simulink model "simModel2020"  (R2023b)
settings: Solver=ode4  StartTime=0  StopTime=360  FixedStep=0.01  RelTol=1e-3
values from neighbouring files (symbols this model uses):
  B747 =     [B747.mat]
undefined symbols (not defined in the file or in its folder): airport, APP, control, Curise, Earth, env, ft, m, navData, navParam, Newton, plotTrack, Raphson, s, TakeOff, WGS84
libraries: aerolibconvert2 x18, simulink x15, sharedtransform x4, aerolibfltsims x3, aerolibatmos2 x2, shared6dof x2, aerolibasang x2, dspsrcs4 x2, aerolibwind2 x2, aerolibanimutils x1, aerolibpropulsion2 x1, aerolibtransform2 x1
(part 4 of 6)

== system simModel2020/AutoPilot/InnerLoopAutopilot/Longitudinal Channel经度通道/AutoThrottle/AT Mode = 3,Throttle Control/Filter1 ==
  x : Inport
  SW_x(k-1) : Inport  Port=2
  time : Inport  Port=3
  Constant : Constant  SampleTime=-1
  Data Type Conversion3 : DataTypeConversion  SaturateOnIntegerOverflow=off  RndMeth=Floor
  Detect Change : simulink/Logic and Bit Operations/Detect Change  vinit=0  OutDataTypeStr=boolean
  Gain : Gain  Gain=0.5
  Math Function : Math  SignedPower=on
  Product : Product
  Product1 : Product
  Subsystem : Subsystem
      mask Display: disp('S/H')
  Sum : Sum  Inputs=|+-
  Sum1 : Sum  Inputs=|++
  Sum2 : Sum  Inputs=+-|
  y : Outport
  wires:
  Product/1 -> Sum1/2
  SW_x(k-1)/1 -> Product/2
  Product1/1 -> Sum1/1
  x/1 -> Product1/1
  Sum1/1 -> Data Type Conversion3/1
  time/1 -> Subsystem/1(In), Sum2/2
  Subsystem/1(" ") -> Sum2/1
  Sum2/1 -> Gain/1
  Gain/1 -> Math Function/1
  Math Function/1 -> Sum/2, Product/1
  Sum/1 -> Product1/2
  Data Type Conversion3/1 -> y/1
  Constant/1 -> Detect Change/1, Sum/1
  Detect Change/1 -> Subsystem/Enable

== system simModel2020/AutoPilot/InnerLoopAutopilot/Longitudinal Channel经度通道/AutoThrottle/AT Mode = 5,Idle/Filter1 ==
  x : Inport
  SW_x(k-1) : Inport  Port=2
  time : Inport  Port=3
  Constant : Constant  SampleTime=-1
  Data Type Conversion3 : DataTypeConversion  SaturateOnIntegerOverflow=off  RndMeth=Floor
  Detect Change : simulink/Logic and Bit Operations/Detect Change  vinit=0  OutDataTypeStr=boolean
  Gain : Gain  Gain=0.5
  Math Function : Math  SignedPower=on
  Product : Product
  Product1 : Product
  Subsystem : Subsystem
      mask Display: disp('S/H')
  Sum : Sum  Inputs=|+-
  Sum1 : Sum  Inputs=|++
  Sum2 : Sum  Inputs=+-|
  y : Outport
  wires:
  Product/1 -> Sum1/2
  SW_x(k-1)/1 -> Product/2
  Product1/1 -> Sum1/1
  x/1 -> Product1/1
  Sum1/1 -> Data Type Conversion3/1
  time/1 -> Subsystem/1(In), Sum2/2
  Subsystem/1(" ") -> Sum2/1
  Sum2/1 -> Gain/1
  Gain/1 -> Math Function/1
  Math Function/1 -> Sum/2, Product/1
  Sum/1 -> Product1/2
  Data Type Conversion3/1 -> y/1
  Constant/1 -> Detect Change/1, Sum/1
  Detect Change/1 -> Subsystem/Enable

== system simModel2020/AutoPilot/InnerLoopAutopilot/Longitudinal Channel经度通道/AutoThrottle/AT Mode = 5,Idle/Rate Limiter Dynamic with External IC and Autoreset for Change in IC ==
  note: Y(k)
  note: U(k)
  up : Inport
  u : Inport  Port=2
  lo : Inport  Port=3
  IC : Inport  Port=4
  Abs : Abs  SaturateOnIntegerOverflow=off
  Delay : Delay  DelayLength=1
  Difference Inputs1 : Sum  Description=Add in CPU  DisableCoverage=on  Inputs=+-  OutDataTypeStr=Inherit: Inherit via back propagation
  Difference Inputs2 : Sum  Description=Add in CPU  OutDataTypeStr=Inherit: Inherit via back propagation
  Saturation Dynamic : Subsystem  mask(Saturation Dynamic){OutMin=[], OutMax=[], OutDataTypeStr=Inherit: Same as second input, OutputDataTypeScalingMode=Same as second input, OutDataType=fixdt(1, 16), OutScaling=2^-10, LockScale=off, RndMeth=Floor, DoSatur=off}
      mask prompts: OutMin "Simulink:masks:OutputMinimum_MP"; OutMax "Simulink:masks:OutputMaximum_MP"; OutDataTypeStr "Simulink:masks:OutputDataType_MP"; OutputDataTypeScalingMode "Simulink:masks:OutputDataTypeMode_MP"; OutDataType "Simulink:masks:OutputDataTypeegFixdt116Fixdtsingle_MP"; OutScaling "Simulink:masks:OutputScalingSlopeEg29OrSlopeBias_MP"; LockScale "Simulink:masks:LockOutputDataTypeAgainstFxpTools_MP"; RndMeth "Simulink:masks:IntegerRoundingMode_MP"; DoSatur "Simulink:masks:SaturateOnIntegerOverflow_MP"
      mask help: Simulink:masks:SaturationDynamic_MD
      mask init: same as simModel2020/AutoPilot/InnerLoopAutopilot/Longitudinal Channel经度通道/AutoThrottle/AT Mode = 0,Recycle/Rate Limiter Dynamic with External IC and Autoreset for Change in IC/Saturation Dynamic
      mask Callback OutDataTypeStr: fixptdialog(gcbh)
      mask TypeOptions OutputDataTypeScalingMode: double | single | int8 | uint8 | int16 | uint16 | int32 | uint32 | Specify via dialog | Same as second input
      mask Callback OutputDataTypeScalingMode: fixptdialog(gcbh)
      mask Callback OutDataType: fixptdialog(gcbh)
      mask TypeOptions RndMeth: Simulink:masks:Ceiling | Simulink:masks:Convergent | Simulink:masks:Floor | Simulink:masks:Nearest | Simulink:masks:Round | Simulink:masks:Simplest | Simulink:masks:Zero
  Subsystem : Subsystem
  Subtract : Sum  Inputs=+-
  Unit Delay Resettable External IC : Subsystem  mask(Unit Delay Resettable External Initial Condition){tsamp=-1}
      mask prompts: tsamp "Simulink:masks:SampleTime_MP"
      mask help: Simulink:masks:UnitDelayResettableExternalInitialCondition_MD
      mask Display: dpoly(1,[1 0],'z')
  delta fall limit : Product  DisableCoverage=on  Inputs=**  OutDataTypeStr=Inherit: Inherit via back propagation  SaturateOnIntegerOverflow=on
  delta rise limit : Product  DisableCoverage=on  Inputs=**  OutDataTypeStr=Inherit: Inherit via back propagation  SaturateOnIntegerOverflow=on
  sample time : SampleTimeMath  DisableCoverage=on  TsampMathOp=Ts Only  weightValue=1
  Y : Outport
  wires:
  Abs/1 -> Subsystem/1(WP Fly)
  Subsystem/1(Just Enab) -> Unit Delay Resettable External IC/2(R)
  Subtract/1 -> Abs/1
  Delay/1 -> Subtract/1
  sample time/1 -> delta fall limit/2, delta rise limit/2
  lo/1 -> delta fall limit/1
  delta rise limit/1 -> Saturation Dynamic/1(up)
  up/1 -> delta rise limit/1
  Difference Inputs2/1 -> Unit Delay Resettable External IC/1(u), Y/1
  Unit Delay Resettable External IC/1(y) -> Difference Inputs1/2, Difference Inputs2/2  "Y(k-1)"
  Saturation Dynamic/1(y) -> Difference Inputs2/1
  delta fall limit/1 -> Saturation Dynamic/3(lo)
  u/1 -> Difference Inputs1/1, sample time/1
  Difference Inputs1/1 -> Saturation Dynamic/2(u)  "( U(k) - Y(k-1) )"
  IC/1 -> Delay/1, Unit Delay Resettable External IC/3(IC), Subtract/2

== system simModel2020/AutoPilot/InnerLoopAutopilot/Longitudinal Channel经度通道/AutoThrottle/Sample(1//z)/Detect Change ==
  note: Edge
  note: U(k)
  U : Inport
  Delay Input1 : UnitDelay  Description=Store in Global RAM  DisableCoverage=on  InitialCondition=vinit  SampleTime=-1  HasFrameUpgradeWarning=on
  FixPt Relational Operator : RelationalOperator  Operator=~=  OutDataTypeStr=boolean  ZeroCross=off  InputSameDT=off
  Y : Outport  InitialOutput=0
  wires:
  FixPt Relational Operator/1 -> Y/1
  Delay Input1/1 -> FixPt Relational Operator/2  "U(k-1)"
  U/1 -> FixPt Relational Operator/1, Delay Input1/1

== system simModel2020/AutoPilot/InnerLoopAutopilot/Longitudinal Channel经度通道/AutoThrottle/Sample(1//z)/Sample and Hold ==
  In : Inport
  Trigger : TriggerPort  TriggerType=either  VariantControl=Variant  ZeroCross=off
  " " : Outport  InitialOutput=initCond
  wires:
  In/1 -> " "/1

== system simModel2020/AutoPilot/InnerLoopAutopilot/Longitudinal Channel经度通道/PitchStyle/Altitude Hold/Filter1 ==
  x : Inport
  SW_x(k-1) : Inport  Port=2
  time : Inport  Port=3
  Constant : Constant  SampleTime=-1
  Data Type Conversion : DataTypeConversion  SaturateOnIntegerOverflow=off  RndMeth=Floor
  Detect Change : simulink/Logic and Bit Operations/Detect Change  vinit=0  OutDataTypeStr=boolean
  Gain : Gain  Gain=0.5
  Math Function : Math  SignedPower=on
  Product : Product
  Product1 : Product
  Subsystem : Subsystem
      mask Display: disp('S/H')
  Sum : Sum  Inputs=|+-
  Sum1 : Sum  Inputs=|++
  Sum2 : Sum  Inputs=+-|
  y : Outport
  wires:
  Product/1 -> Sum1/2
  SW_x(k-1)/1 -> Product/2
  Product1/1 -> Sum1/1
  x/1 -> Product1/1
  Sum1/1 -> Data Type Conversion/1
  time/1 -> Subsystem/1(In), Sum2/2
  Subsystem/1(" ") -> Sum2/1
  Sum2/1 -> Gain/1
  Gain/1 -> Math Function/1
  Math Function/1 -> Product/1, Sum/2
  Sum/1 -> Product1/2
  Data Type Conversion/1 -> y/1
  Constant/1 -> Sum/1, Detect Change/1
  Detect Change/1 -> Subsystem/Enable

== system simModel2020/AutoPilot/InnerLoopAutopilot/Longitudinal Channel经度通道/PitchStyle/IAS_Control_dE/Filter2 ==
  x : Inport
  SW_x(k-1) : Inport  Port=2
  time : Inport  Port=3
  Constant : Constant  SampleTime=-1
  Data Type Conversion3 : DataTypeConversion  SaturateOnIntegerOverflow=off  RndMeth=Floor
  Detect Change : simulink/Logic and Bit Operations/Detect Change  vinit=0  OutDataTypeStr=boolean
  Gain : Gain  Gain=0.5
  Math Function : Math  SignedPower=on
  Product : Product
  Product1 : Product
  Subsystem : Subsystem
      mask Display: disp('S/H')
  Sum : Sum  Inputs=|+-
  Sum1 : Sum  Inputs=|++
  Sum2 : Sum  Inputs=+-|
  y : Outport
  wires:
  Product/1 -> Sum1/2
  SW_x(k-1)/1 -> Product/2
  Product1/1 -> Sum1/1
  x/1 -> Product1/1
  Sum1/1 -> Data Type Conversion3/1
  time/1 -> Subsystem/1(In), Sum2/2
  Subsystem/1(" ") -> Sum2/1
  Sum2/1 -> Gain/1
  Gain/1 -> Math Function/1
  Math Function/1 -> Sum/2, Product/1
  Sum/1 -> Product1/2
  Data Type Conversion3/1 -> y/1
  Constant/1 -> Detect Change/1, Sum/1
  Detect Change/1 -> Subsystem/Enable

== system simModel2020/AutoPilot/InnerLoopAutopilot/Longitudinal Channel经度通道/PitchStyle/Pitch Control/Compute Feed Forward ==
  dEFFGain : Inport
  Roll : Inport  Port=2
  Add5 : Sum  Inputs=+-  OutDataTypeStr=single
  Constant2 : Constant  OutDataTypeStr=single
      settings: AttributesFormatString=%<Value>
  Constant4 : Constant  OutDataTypeStr=single
      settings: AttributesFormatString=%<Value>
  Product : Product  Inputs=*/  RndMeth=Zero
  Product1 : Product  RndMeth=Zero
  Saturation : Saturate  UpperLimit=pi/3  LowerLimit=-pi/3  OutDataTypeStr=double
  Trigonometric Function : Trigonometry  Operator=cos
  FF : Outport
  wires:
  Product/1 -> Add5/1
  Constant4/1 -> Product/1
  Roll/1 -> Saturation/1
  Trigonometric Function/1 -> Product/2
  Constant2/1 -> Add5/2
  Product1/1 -> FF/1
  Add5/1 -> Product1/2
  Saturation/1 -> Trigonometric Function/1
  dEFFGain/1 -> Product1/1

== system simModel2020/AutoPilot/InnerLoopAutopilot/Longitudinal Channel经度通道/PitchStyle/Pitch Control/Filter2 ==
  x : Inport
  SW_x(k-1) : Inport  Port=2
  time : Inport  Port=3
  Constant : Constant  SampleTime=-1
  Data Type Conversion3 : DataTypeConversion  SaturateOnIntegerOverflow=off  RndMeth=Floor
  Detect Change : simulink/Logic and Bit Operations/Detect Change  vinit=0  OutDataTypeStr=boolean
  Gain : Gain  Gain=0.5
  Math Function : Math  SignedPower=on
  Product : Product
  Product1 : Product
  Subsystem : Subsystem
      mask Display: disp('S/H')
  Sum : Sum  Inputs=|+-
  Sum1 : Sum  Inputs=|++
  Sum2 : Sum  Inputs=+-|
  y : Outport
  wires:
  Product/1 -> Sum1/2
  SW_x(k-1)/1 -> Product/2
  Product1/1 -> Sum1/1
  x/1 -> Product1/1
  Sum1/1 -> Data Type Conversion3/1
  time/1 -> Subsystem/1(In), Sum2/2
  Subsystem/1(" ") -> Sum2/1
  Sum2/1 -> Gain/1
  Gain/1 -> Math Function/1
  Math Function/1 -> Sum/2, Product/1
  Sum/1 -> Product1/2
  Data Type Conversion3/1 -> y/1
  Constant/1 -> Detect Change/1, Sum/1
  Detect Change/1 -> Subsystem/Enable

== system simModel2020/AutoPilot/InnerLoopAutopilot/Longitudinal Channel经度通道/PitchStyle/Rate Limiter Dynamic/Rate Limiter Dynamic with External IC and Autoreset for Change in IC1 ==
  note: U(k)
  note: Y(k)
  up : Inport
  u : Inport  Port=2
  lo : Inport  Port=3
  IC : Inport  Port=4
  Abs : Abs  SaturateOnIntegerOverflow=off
  Delay : Delay  DelayLength=1
  Difference Inputs1 : Sum  Description=Add in CPU  DisableCoverage=on  Inputs=+-  OutDataTypeStr=Inherit: Inherit via back propagation
  Difference Inputs2 : Sum  Description=Add in CPU  OutDataTypeStr=Inherit: Inherit via back propagation
  Saturation Dynamic : Subsystem  mask(Saturation Dynamic){OutMin=[], OutMax=[], OutDataTypeStr=Inherit: Same as second input, OutputDataTypeScalingMode=Same as second input, OutDataType=fixdt(1, 16), OutScaling=2^-10, LockScale=off, RndMeth=Floor, DoSatur=off}
      mask prompts: OutMin "Simulink:masks:OutputMinimum_MP"; OutMax "Simulink:masks:OutputMaximum_MP"; OutDataTypeStr "Simulink:masks:OutputDataType_MP"; OutputDataTypeScalingMode "Simulink:masks:OutputDataTypeMode_MP"; OutDataType "Simulink:masks:OutputDataTypeegFixdt116Fixdtsingle_MP"; OutScaling "Simulink:masks:OutputScalingSlopeEg29OrSlopeBias_MP"; LockScale "Simulink:masks:LockOutputDataTypeAgainstFxpTools_MP"; RndMeth "Simulink:masks:IntegerRoundingMode_MP"; DoSatur "Simulink:masks:SaturateOnIntegerOverflow_MP"
      mask help: Simulink:masks:SaturationDynamic_MD
      mask init: same as simModel2020/AutoPilot/InnerLoopAutopilot/Longitudinal Channel经度通道/AutoThrottle/AT Mode = 0,Recycle/Rate Limiter Dynamic with External IC and Autoreset for Change in IC/Saturation Dynamic
      mask Callback OutDataTypeStr: fixptdialog(gcbh)
      mask TypeOptions OutputDataTypeScalingMode: double | single | int8 | uint8 | int16 | uint16 | int32 | uint32 | Specify via dialog | Same as second input
      mask Callback OutputDataTypeScalingMode: fixptdialog(gcbh)
      mask Callback OutDataType: fixptdialog(gcbh)
      mask TypeOptions RndMeth: Simulink:masks:Ceiling | Simulink:masks:Convergent | Simulink:masks:Floor | Simulink:masks:Nearest | Simulink:masks:Round | Simulink:masks:Simplest | Simulink:masks:Zero
  Subsystem : Subsystem
  Subtract : Sum  Inputs=+-
  Unit Delay Resettable External IC : Subsystem  mask(Unit Delay Resettable External Initial Condition){tsamp=-1}
      mask prompts: tsamp "Simulink:masks:SampleTime_MP"
      mask help: Simulink:masks:UnitDelayResettableExternalInitialCondition_MD
      mask Display: dpoly(1,[1 0],'z')
  Weighted Sample Time : SampleTimeMath  TsampMathOp=Ts Only
  delta fall limit : Product  DisableCoverage=on  Inputs=**  OutDataTypeStr=Inherit: Inherit via back propagation  SaturateOnIntegerOverflow=on
  delta rise limit : Product  DisableCoverage=on  Inputs=**  OutDataTypeStr=Inherit: Inherit via back propagation  SaturateOnIntegerOverflow=on
  Y : Outport
  wires:
  IC/1 -> Subtract/2, Unit Delay Resettable External IC/3(IC), Delay/1
  Difference Inputs1/1 -> Saturation Dynamic/2(u)  "( U(k) - Y(k-1) )"
  u/1 -> Difference Inputs1/1, Weighted Sample Time/1
  delta fall limit/1 -> Saturation Dynamic/3(lo)
  Saturation Dynamic/1(y) -> Difference Inputs2/1
  Unit Delay Resettable External IC/1(y) -> Difference Inputs2/2, Difference Inputs1/2  "Y(k-1)"
  Difference Inputs2/1 -> Y/1, Unit Delay Resettable External IC/1(u)
  up/1 -> delta rise limit/1
  delta rise limit/1 -> Saturation Dynamic/1(up)
  lo/1 -> delta fall limit/1
  Weighted Sample Time/1 -> delta rise limit/2, delta fall limit/2
  Delay/1 -> Subtract/1
  Subtract/1 -> Abs/1
  Subsystem/1(Just Enab) -> Unit Delay Resettable External IC/2(R)
  Abs/1 -> Subsystem/1(WP Fly)

== system simModel2020/AutoPilot/InnerLoopAutopilot/Longitudinal Channel经度通道/PitchStyle/Rate Limiter Dynamic/Sample(1//z) ==
  <Test> : Inport
  x : Inport  Port=2
  Detect Change : Subsystem  mask(Detect Change){vinit=0, InputProcessing=Elements as channels (sample based), OutDataTypeStr=boolean}
      mask prompts: vinit "Simulink:masks:InitialCondition_MP"; InputProcessing "Simulink:masks:InputProcessing_MP"; OutDataTypeStr "Simulink:masks:OutputDataType_MP"
      mask help: Simulink:masks:DetectChange_MD
      mask init:
      | initDetectBlocks();
      mask TypeOptions InputProcessing: Simulink:masks:ColumnsAsChannelsFrameBased | Simulink:masks:ElementsAsChannelsSampleBased
      mask TypeOptions OutDataTypeStr: Simulink:masks:uint8 | Simulink:masks:boolean
      mask Display: fprintf('U ~= U/z')
  Sample and Hold : Subsystem  TreatAsAtomicUnit=on  mask(Sample and Hold){trig=Either edge, initCond=0, latchinput=off}
      mask prompts: trig "Trigger type:"; initCond "Initial condition:"; latchinput "Latch (buffer) input"
      mask help: Sample and hold the input signal. If Latch (buffer) input is selected, then this block produces the value of the input from the previous time step.
      mask init: same as simModel2020/AutoPilot/InnerLoopAutopilot/Latitudinal Channel维度通道/Sample(1//z)/Sample and Hold
      mask Help: eval('blocksethelp');
      mask TypeOptions trig: Rising edge | Falling edge | Either edge
      mask Display: disp('S/H')
  y : Outport
  wires:
  <Test>/1 -> Detect Change/1(U)
  Detect Change/1(Y) -> Sample and Hold/Trigger
  x/1 -> Sample and Hold/1(In)
  Sample and Hold/1(" ") -> y/1

== system simModel2020/AutoPilot/InnerLoopAutopilot/Longitudinal Channel经度通道/PitchStyle/Rate Limiter Dynamic1/Rate Limiter Dynamic with External IC and Autoreset for Change in IC ==
  note: Y(k)
  note: U(k)
  up : Inport
  u : Inport  Port=2
  lo : Inport  Port=3
  IC : Inport  Port=4
  Abs : Abs  SaturateOnIntegerOverflow=off
  Delay : Delay  DelayLength=1
  Difference Inputs1 : Sum  Description=Add in CPU  DisableCoverage=on  Inputs=+-  OutDataTypeStr=Inherit: Inherit via back propagation
  Difference Inputs2 : Sum  Description=Add in CPU  OutDataTypeStr=Inherit: Inherit via back propagation
  Saturation Dynamic : Subsystem  mask(Saturation Dynamic){OutMin=[], OutMax=[], OutDataTypeStr=Inherit: Same as second input, OutputDataTypeScalingMode=Same as second input, OutDataType=fixdt(1, 16), OutScaling=2^-10, LockScale=off, RndMeth=Floor, DoSatur=off}
      mask prompts: OutMin "Simulink:masks:OutputMinimum_MP"; OutMax "Simulink:masks:OutputMaximum_MP"; OutDataTypeStr "Simulink:masks:OutputDataType_MP"; OutputDataTypeScalingMode "Simulink:masks:OutputDataTypeMode_MP"; OutDataType "Simulink:masks:OutputDataTypeegFixdt116Fixdtsingle_MP"; OutScaling "Simulink:masks:OutputScalingSlopeEg29OrSlopeBias_MP"; LockScale "Simulink:masks:LockOutputDataTypeAgainstFxpTools_MP"; RndMeth "Simulink:masks:IntegerRoundingMode_MP"; DoSatur "Simulink:masks:SaturateOnIntegerOverflow_MP"
      mask help: Simulink:masks:SaturationDynamic_MD
      mask init: same as simModel2020/AutoPilot/InnerLoopAutopilot/Longitudinal Channel经度通道/AutoThrottle/AT Mode = 0,Recycle/Rate Limiter Dynamic with External IC and Autoreset for Change in IC/Saturation Dynamic
      mask Callback OutDataTypeStr: fixptdialog(gcbh)
      mask TypeOptions OutputDataTypeScalingMode: double | single | int8 | uint8 | int16 | uint16 | int32 | uint32 | Specify via dialog | Same as second input
      mask Callback OutputDataTypeScalingMode: fixptdialog(gcbh)
      mask Callback OutDataType: fixptdialog(gcbh)
      mask TypeOptions RndMeth: Simulink:masks:Ceiling | Simulink:masks:Convergent | Simulink:masks:Floor | Simulink:masks:Nearest | Simulink:masks:Round | Simulink:masks:Simplest | Simulink:masks:Zero
  Subsystem : Subsystem
  Subtract : Sum  Inputs=+-
  Unit Delay Resettable External IC : Subsystem  mask(Unit Delay Resettable External Initial Condition){tsamp=-1}
      mask prompts: tsamp "Simulink:masks:SampleTime_MP"
      mask help: Simulink:masks:UnitDelayResettableExternalInitialCondition_MD
      mask Display: dpoly(1,[1 0],'z')
  Weighted Sample Time : SampleTimeMath  TsampMathOp=Ts Only  OutDataTypeStr=Inherit: Inherit via back propagation
  delta fall limit : Product  DisableCoverage=on  Inputs=**  OutDataTypeStr=Inherit: Inherit via back propagation  SaturateOnIntegerOverflow=on
  delta rise limit : Product  DisableCoverage=on  Inputs=**  OutDataTypeStr=Inherit: Inherit via back propagation  SaturateOnIntegerOverflow=on
  Y : Outport
  wires:
  Abs/1 -> Subsystem/1(WP Fly)
  Subsystem/1(Just Enab) -> Unit Delay Resettable External IC/2(R)
  Subtract/1 -> Abs/1
  Delay/1 -> Subtract/1
  Weighted Sample Time/1 -> delta fall limit/2, delta rise limit/2
  lo/1 -> delta fall limit/1
  delta rise limit/1 -> Saturation Dynamic/1(up)
  up/1 -> delta rise limit/1
  Difference Inputs2/1 -> Unit Delay Resettable External IC/1(u), Y/1
  Unit Delay Resettable External IC/1(y) -> Difference Inputs1/2, Difference Inputs2/2  "Y(k-1)"
  Saturation Dynamic/1(y) -> Difference Inputs2/1
  delta fall limit/1 -> Saturation Dynamic/3(lo)
  u/1 -> Weighted Sample Time/1, Difference Inputs1/1
  Difference Inputs1/1 -> Saturation Dynamic/2(u)  "( U(k) - Y(k-1) )"
  IC/1 -> Delay/1, Unit Delay Resettable External IC/3(IC), Subtract/2

== system simModel2020/AutoPilot/InnerLoopAutopilot/Longitudinal Channel经度通道/PitchStyle/Rate Limiter Dynamic1/Sample(1//z) ==
  <Test> : Inport
  x : Inport  Port=2
  Detect Change : Subsystem  mask(Detect Change){vinit=0, InputProcessing=Elements as channels (sample based), OutDataTypeStr=boolean}
      mask prompts: vinit "Simulink:masks:InitialCondition_MP"; InputProcessing "Simulink:masks:InputProcessing_MP"; OutDataTypeStr "Simulink:masks:OutputDataType_MP"
      mask help: Simulink:masks:DetectChange_MD
      mask init:
      | initDetectBlocks();
      mask TypeOptions InputProcessing: Simulink:masks:ColumnsAsChannelsFrameBased | Simulink:masks:ElementsAsChannelsSampleBased
      mask TypeOptions OutDataTypeStr: Simulink:masks:uint8 | Simulink:masks:boolean
      mask Display: fprintf('U ~= U/z')
  Sample and Hold : Subsystem  TreatAsAtomicUnit=on  mask(Sample and Hold){trig=Either edge, initCond=0, latchinput=off}
      mask prompts: trig "Trigger type:"; initCond "Initial condition:"; latchinput "Latch (buffer) input"
      mask help: Sample and hold the input signal. If Latch (buffer) input is selected, then this block produces the value of the input from the previous time step.
      mask init: same as simModel2020/AutoPilot/InnerLoopAutopilot/Latitudinal Channel维度通道/Sample(1//z)/Sample and Hold
      mask Help: eval('blocksethelp');
      mask TypeOptions trig: Rising edge | Falling edge | Either edge
      mask Display: disp('S/H')
  y : Outport
  wires:
  <Test>/1 -> Detect Change/1(U)
  Detect Change/1(Y) -> Sample and Hold/Trigger
  x/1 -> Sample and Hold/1(In)
  Sample and Hold/1(" ") -> y/1

== system simModel2020/AutoPilot/InnerLoopAutopilot/Longitudinal Channel经度通道/PitchStyle/Sample(1//z)/Detect Change ==
  note: Edge
  note: U(k)
  U : Inport
  Delay Input1 : UnitDelay  Description=Store in Global RAM  DisableCoverage=on  InitialCondition=vinit  SampleTime=-1  HasFrameUpgradeWarning=on
  FixPt Relational Operator : RelationalOperator  Operator=~=  OutDataTypeStr=boolean  ZeroCross=off  InputSameDT=off
  Y : Outport  InitialOutput=0
  wires:
  FixPt Relational Operator/1 -> Y/1
  Delay Input1/1 -> FixPt Relational Operator/2  "U(k-1)"
  U/1 -> FixPt Relational Operator/1, Delay Input1/1

== system simModel2020/AutoPilot/InnerLoopAutopilot/Longitudinal Channel经度通道/PitchStyle/Sample(1//z)/Sample and Hold ==
  In : Inport
  Trigger : TriggerPort  TriggerType=either  VariantControl=Variant  ZeroCross=off
  " " : Outport  InitialOutput=initCond
  wires:
  In/1 -> " "/1

== system simModel2020/AutoPilot/InnerLoopAutopilot/Longitudinal Channel经度通道/PitchStyle/Sample(1//z)1/Detect Change ==
  note: Edge
  note: U(k)
  U : Inport
  Delay Input1 : UnitDelay  Description=Store in Global RAM  DisableCoverage=on  InitialCondition=vinit  SampleTime=-1  HasFrameUpgradeWarning=on
  FixPt Relational Operator : RelationalOperator  Operator=~=  OutDataTypeStr=boolean  ZeroCross=off  InputSameDT=off
  Y : Outport  InitialOutput=0
  wires:
  FixPt Relational Operator/1 -> Y/1
  Delay Input1/1 -> FixPt Relational Operator/2  "U(k-1)"
  U/1 -> FixPt Relational Operator/1, Delay Input1/1

== system simModel2020/AutoPilot/InnerLoopAutopilot/Longitudinal Channel经度通道/PitchStyle/Sample(1//z)1/Sample and Hold ==
  In : Inport
  Trigger : TriggerPort  TriggerType=either  VariantControl=Variant  ZeroCross=off
  " " : Outport  InitialOutput=initCond
  wires:
  In/1 -> " "/1

== system simModel2020/AutoPilot/InnerLoopAutopilot/Longitudinal Channel经度通道/PitchStyle/Vtertical Speed Control/Filter1 ==
  x : Inport
  SW_x(k-1) : Inport  Port=2
  time : Inport  Port=3
  Constant : Constant  SampleTime=-1
  Data Type Conversion3 : DataTypeConversion  SaturateOnIntegerOverflow=off  RndMeth=Floor
  Detect Change : simulink/Logic and Bit Operations/Detect Change  vinit=0  OutDataTypeStr=boolean
  Gain : Gain  Gain=0.5
  Math Function : Math  SignedPower=on
  Product : Product
  Product1 : Product
  Subsystem : Subsystem
      mask Display: disp('S/H')
  Sum : Sum  Inputs=|+-
  Sum1 : Sum  Inputs=|++
  Sum2 : Sum  Inputs=+-|
  y : Outport
  wires:
  Product/1 -> Sum1/2
  SW_x(k-1)/1 -> Product/2
  Product1/1 -> Sum1/1
  x/1 -> Product1/1
  Sum1/1 -> Data Type Conversion3/1
  time/1 -> Subsystem/1(In), Sum2/2
  Subsystem/1(" ") -> Sum2/1
  Sum2/1 -> Gain/1
  Gain/1 -> Math Function/1
  Math Function/1 -> Sum/2, Product/1
  Sum/1 -> Product1/2
  Data Type Conversion3/1 -> y/1
  Constant/1 -> Detect Change/1, Sum/1
  Detect Change/1 -> Subsystem/Enable

== system simModel2020/PlantModel/B747 Dynamics动力学参数计算/Forces and Moments动力学计算/Compute Air Data迎角侧滑角计算/Dynamic Pressure动压/dot ==
  V : Inport
  Demux1 : Demux  Outputs=3
  Product : Product  RndMeth=Zero
  Product1 : Product  RndMeth=Zero
  Product2 : Product  RndMeth=Zero
  Sum : Sum  Inputs=+++
  dot : Outport
  wires:
  Product2/1 -> Sum/3
  Demux1/3 -> Product2/2, Product2/1
  Product/1 -> Sum/1
  Product1/1 -> Sum/2
  Sum/1 -> dot/1
  V/1 -> Demux1/1
  Demux1/1 -> Product/2, Product/1
  Demux1/2 -> Product1/1, Product1/2

== system simModel2020/PlantModel/B747 Dynamics动力学参数计算/Forces and Moments动力学计算/Compute Body Frame Forces and Moments气动力和力矩/Rotate FM to body frame/Rotate Forces ==
  F_w : Inport
  alpha_beta : Inport  Port=2
  Math Function : Math  Operator=transpose  SignedPower=on
  Product2 : Product  Multiplication=Matrix(*)  SaturateOnIntegerOverflow=on  OutDataTypeStr=Inherit: Same as first input
  RB2W : Subsystem
  F_b : Outport  PortDimensions=3
  wires:
  F_w/1 -> Product2/2
  Product2/1 -> F_b/1
  alpha_beta/1 -> RB2W/1(aoa beta)
  Math Function/1 -> Product2/1
  RB2W/1(Rw2b) -> Math Function/1

== system simModel2020/PlantModel/B747 Dynamics动力学参数计算/Forces and Moments动力学计算/Compute Body Frame Forces and Moments气动力和力矩/Rotate FM to body frame/Rotate Moments ==
  alpha_beta : Inport
  M_w : Inport  Port=2
  Math Function : Math  Operator=transpose  SignedPower=on
  Product2 : Product  Multiplication=Matrix(*)  SaturateOnIntegerOverflow=on  OutDataTypeStr=Inherit: Same as first input
  RB2W : Subsystem
  M_b : Outport  PortDimensions=3
  wires:
  RB2W/1(Rw2b) -> Math Function/1
  alpha_beta/1 -> RB2W/1(aoa beta)
  Product2/1 -> M_b/1
  M_w/1 -> Product2/2
  Math Function/1 -> Product2/1

== system simModel2020/PlantModel/B747 Dynamics动力学参数计算/Forces and Moments动力学计算/Compute Body Frame Forces and Moments气动力和力矩/Wind frame F& M 气动力计算/Get Forces and Moments ==
  note: S为机翼参考面积
  note: chord为c_A平均几何弦长
  note: span=b，机翼展长
  note: q为动压
  note: 升力
  note: 侧力
  note: 阻力
  note: 俯仰力矩
  note: 滚转力矩
  note: 偏航力矩
  note: chord为c_A平均几何弦长
  Airdata : Inport
  AeroCoeffs : Inport  Port=2
  Bus Selector : BusSelector  OutputSignals=signal2.CD,signal1.CY,signal2.CL
  Bus Selector3 : BusSelector  OutputSignals=signal1.Cl,signal1.Cn
  Bus Selector4 : BusSelector  OutputSignals=signal2.Cm
  Bus Selector5 : BusSelector  OutputSignals=q
  Fx_a(Drag) : Product  Inputs=**  SaturateOnIntegerOverflow=on  OutDataTypeStr=Inherit: Same as first input
  Fy_a(Side) : Product  SaturateOnIntegerOverflow=on  OutDataTypeStr=Inherit: Same as first input
  Fz_a(Lift) : Product  SaturateOnIntegerOverflow=on  OutDataTypeStr=Inherit: Same as first input
  Mux : Mux  Inputs=6
  Mx_a : Product  Inputs=3  SaturateOnIntegerOverflow=on  OutDataTypeStr=Inherit: Same as first input
  My_a : Product  Inputs=3  SaturateOnIntegerOverflow=on  OutDataTypeStr=Inherit: Same as first input
  Mz_a : Product  Inputs=3  SaturateOnIntegerOverflow=on  OutDataTypeStr=Inherit: Same as first input
  Product1 : Product  Inputs=3  SaturateOnIntegerOverflow=on  OutDataTypeStr=Inherit: Same as first input
  chord : Constant  Value=B747.geometry.chord  VectorParams1D=off
      settings: AttributesFormatString=%<Value>
  span : Constant  Value=B747.geometry.span  VectorParams1D=off
      settings: AttributesFormatString=%<Value>
  span1 : Constant  Value=B747.geometry.span  VectorParams1D=off
      settings: AttributesFormatString=%<Value>
  span2 : Constant  Value=B747.geometry.chord  VectorParams1D=off
      settings: AttributesFormatString=%<Value>
  FM_w : Outport
  wires:
  Mx_a/1 -> Mux/4  "Mx_a"
  Bus Selector/2 -> Fy_a(Side)/1  "<CY>"
  Bus Selector4/1 -> My_a/1  "<Cm>"
  span2/1 -> Product1/3
  Fx_a(Drag)/1 -> Mux/1  "Fx_a"
  Bus Selector/1 -> Fx_a(Drag)/1  "<CD>"
  AeroCoeffs/1 -> Bus Selector/1, Bus Selector4/1, Bus Selector3/1
  My_a/1 -> Mux/5  "My_a"
  Fz_a(Lift)/1 -> Mux/3  "Fz_a"
  Mz_a/1 -> Mux/6  "Mz_a"
  Airdata/1 -> Bus Selector5/1
  chord/1 -> My_a/3
  span/1 -> Mx_a/3, Mz_a/3
  Fy_a(Side)/1 -> Mux/2  "Fy_a"
  Mux/1 -> FM_w/1
  Bus Selector3/2 -> Mz_a/1  "<Cn>"
  Bus Selector/3 -> Fz_a(Lift)/1  "<CL>"
  Product1/1 -> Fx_a(Drag)/2, Fy_a(Side)/2, Fz_a(Lift)/2, Mx_a/2, My_a/2, Mz_a/2  "qS"
  span1/1 -> Product1/2
  Bus Selector3/1 -> Mx_a/1  "<Cl>"
  Bus Selector5/1 -> Product1/1  "<q>"

== system simModel2020/PlantModel/B747 Dynamics动力学参数计算/Forces and Moments动力学计算/Compute Body Frame Forces and Moments气动力和力矩/Wind frame F& M 气动力计算/Lateral Channel ==
  note: 偏航力矩系数
  note: 滚转力矩系数
  note: 侧力系数
  beta : Inport
  Airspeed : Inport  Port=2
  dA : Inport  Port=3
  dR : Inport  Port=4
  p,q,r : Inport  Port=5
  Deviation On : Inport  Port=6
  Bus Creator : BusCreator  Inputs=3
  CY : Subsystem
  Cl : Subsystem
  Cn : Subsystem
  Lateral : Outport
  wires:
  Cl/1(Cl) -> Bus Creator/2  "Cl"
  p,q,r/1 -> Cn/4(p,q,r), Cl/4(p,q,r)
  Airspeed/1 -> Cn/5(Airspeed), Cl/5(Airspeed)
  dR/1 -> CY/2(dR), Cl/3(dR), Cn/3(Dr)
  dA/1 -> Cl/2(dA), Cn/2(dA)
  beta/1 -> CY/1(beta), Cl/1(beta), Cn/1(beta)
  Cn/1(Cn) -> Bus Creator/3  "Cn"
  CY/1(CY) -> Bus Creator/1  "CY"
  Bus Creator/1 -> Lateral/1
  Deviation On/1 -> Cl/6(Deviation On)

== system simModel2020/PlantModel/B747 Dynamics动力学参数计算/Forces and Moments动力学计算/Compute Body Frame Forces and Moments气动力和力矩/Wind frame F& M 气动力计算/Longitudinal Channel ==
  note: 俯仰力矩系数
  note: 升力系数
  note: 阻力系数
  alpha : Inport
  Airpseed : Inport  Port=2
  dE : Inport  Port=3
  dF : Inport  Port=4
  p,q,r : Inport  Port=5
  Deviation On : Inport  Port=6
  Bus Creator : BusCreator  Inputs=3
  CD : Subsystem
  CL : Subsystem
  Cm : Subsystem
  Y-down : Gain  Gain=-1  SaturateOnIntegerOverflow=on  OutDataTypeStr=Inherit: Same as input  ParamDataTypeStr=Inherit: Same as input
      settings: AttributesFormatString=%<Gain>
  Longitudinal : Outport
  wires:
  Airpseed/1 -> Cm/4(Airspeed), CL/6(Airspeed)
  p,q,r/1 -> Cm/3(p,q,r), CL/5(p,q,r)
  dF/1 -> CL/4(dF), Cm/6(dF)
  Bus Creator/1 -> Longitudinal/1
  Cm/1(Cm) -> Bus Creator/3  "Cm"
  CL/1(CL) -> Y-down/1
  dE/1 -> Cm/2(dE), CL/3(dE)
  Y-down/1 -> Bus Creator/2  "CL"
  CD/1(CD) -> Bus Creator/1  "CD"
  alpha/1 -> CD/1(alpha), Cm/1(alpha), CL/2(alpha)
  Deviation On/1 -> Cm/5(Deviation On), CL/1(Deviation On), CD/2(Deviation On)

== system simModel2020/PlantModel/B747 Dynamics动力学参数计算/Forces and Moments动力学计算/Engine Model/ Turbofan Engine System/N1 caculation 包含大气参数计算 ==
  sqrt(theta) : Inport
  Throttle_cmd : Inport  Port=2
  Altitude : Inport  Port=3
  Mach : Inport  Port=4
  CN1_PLA(Mach,IAP) : Lookup_n-D  NumberOfTableDimensions=3  BreakpointsForDimension1=[0 0.4 0.5 0.6 0.7 0.8 0.9 1.0]  BreakpointsForDimension2=[0 0.9]  BreakpointsForDimension3=[1 22.5]  Table=CN1  InternalRulePriority=Speed  RndMeth=Simplest
      mask init:
      | CN1=cat(3,[20 84;67 96.5;72 102;82 104;90 107;94 108;104 109.5;109 111],[43 79;
      |     56.5 97;64 102.5;76 104.5;88.5 107;95 108;105 109.5;109 111]);
      settings: InputPortMap=u0,u1,u2
  ISA Atmosphere Model大气参数计算 : aerolibatmos2/ISA Atmosphere Model  useExtended=off  action=Warning  custom=off  viscosityOut=off  g=9.80665  gamma=1.4  R=287.0531  L=0.0065  h_trop=11000  h_strat=20000  rho0=1.225  P0=101325  T0=288.15  h0=0
  Math Function : Math  Operator=reciprocal  SignedPower=on
  P0 : Gain  Gain=101325
  Product : Product
  Saturation1 : Saturate  UpperLimit=100  LowerLimit=0
  Terminator : Terminator
  Terminator1 : Terminator
  Terminator2 : Terminator
  N1(%) : Outport
  wires:
  Math Function/1 -> P0/1
  ISA Atmosphere Model大气参数计算/1 -> Terminator/1
  P0/1 -> CN1_PLA(Mach,IAP)/3  "IAP=P0/P"
  ISA Atmosphere Model大气参数计算/3 -> Math Function/1
  ISA Atmosphere Model大气参数计算/2 -> Terminator1/1
  ISA Atmosphere Model大气参数计算/4 -> Terminator2/1
  CN1_PLA(Mach,IAP)/1 -> Product/2
  sqrt(theta)/1 -> Product/1
  Altitude/1 -> ISA Atmosphere Model大气参数计算/1
  Throttle_cmd/1 -> CN1_PLA(Mach,IAP)/1
  Mach/1 -> CN1_PLA(Mach,IAP)/2
  Product/1 -> Saturation1/1
  Saturation1/1 -> N1(%)/1  "F"

== system simModel2020/PlantModel/B747 Dynamics动力学参数计算/Forces and Moments动力学计算/Engine Model/ Turbofan Engine System/Subsystem ==
  thrust : Inport
  sqrt(theta) : Inport  Port=2
  delta : Inport  Port=3
  Fmax1 : Constant  Value=1/Fmax
  Product2 : Product  Inputs=*/**  InputSameDT=on  SaturateOnIntegerOverflow=on  OutDataTypeStr=Inherit: Same as first input
  Product5 : Product  Inputs=**/  InputSameDT=on  SaturateOnIntegerOverflow=on  OutDataTypeStr=Inherit: Same as first input
  Tau(Thrust) : Lookup_n-D  NumberOfTableDimensions=1  BreakpointsForDimension1=[0.0:0.04:1.0]  IndexSearchMethod=Evenly spaced points  Table=Tau  ExtrapMethod=Clip
      mask init:
      | Tau=[5.18 4.14 3.32 2.68 2.19 1.83 1.56 1.33 1.23 1.15 1.1 1.06 1.04 1.03 1.02 1.01	1 1 1 1 1 1 1 1 1 1];
  "tau " : Constant  Value=tau
  tau : Outport
  wires:
  Fmax1/1 -> Product5/1
  "tau "/1 -> Product2/3
  delta/1 -> Product5/3, Product2/4
  sqrt(theta)/1 -> Product2/2
  Product2/1 -> tau/1
  Tau(Thrust)/1 -> Product2/1
  Product5/1 -> Tau(Thrust)/1
  thrust/1 -> Product5/2

== system simModel2020/PlantModel/B747 Dynamics动力学参数计算/Forces and Moments动力学计算/Engine Model/ Turbofan Engine System/Transfer function ==
  tau : Inport
  T_tgt : Inport  Port=2
  IC2 : Constant  Value=IC
  Integrator1 : Integrator  InitialConditionSource=external
  Product5 : Product  Inputs=*/  InputSameDT=on  SaturateOnIntegerOverflow=on  OutDataTypeStr=Inherit: Same as first input
  Saturation1 : Saturate  UpperLimit=Fmax  LowerLimit=0
  Sum1 : Sum  Inputs=|+-  InputSameDT=on  SaturateOnIntegerOverflow=on  OutDataTypeStr=Inherit: Same as first input
  T_out : Outport
  wires:
  Product5/1 -> Integrator1/1
  Integrator1/1 -> Sum1/2, T_out/1
  Sum1/1 -> Product5/1
  IC2/1 -> Integrator1/2
  tau/1 -> Product5/2
  Saturation1/1 -> Sum1/1  "F"
  T_tgt/1 -> Saturation1/1

== system simModel2020/AutoPilot/InnerLoopAutopilot/Longitudinal Channel经度通道/AutoThrottle/AT Mode = 0,Recycle/Filter1/Subsystem ==
  In : Inport
  Enable : EnablePort  StatesWhenEnabling=reset
  " " : Outport  InitialOutput=0
  wires:
  In/1 -> " "/1

== system simModel2020/AutoPilot/InnerLoopAutopilot/Longitudinal Channel经度通道/AutoThrottle/AT Mode = 0,Recycle/Rate Limiter Dynamic with External IC and Autoreset for Change in IC/Saturation Dynamic ==
  up : Inport
  u : Inport  Port=2
  lo : Inport  Port=3
  Data Type Duplicate : DataTypeDuplicate  DisableCoverage=on
  Data Type Propagation : S-Function  FunctionName=sfix_dtprop  Parameters=14,PropDataTypeMode,(getdatatypespecs(PropDataType,PropScaling,DblOver,0, 0, PropDataTypeMode, PropScalingMode)),IfRefDouble,IfRefSingle,IsSigned,NumBitsBase,NumBitsMult,NumBitsAdd,(sort(reshape(round(NumBitsAllowFinal), prod(size(NumBitsAllowFinal)),1))),PropScalingMode,ValuesUsedBestPrec,SlopeBase,SlopeMult,SlopeAdd,BiasBase,BiasMult,BiasAdd,DblOver  SFunctionDeploymentMode=off  EnableBusSupport=off  mask(Data Type Propagation){PropDataTypeMode=Inherit via propagation rule, PropDataType=fixdt(1, 16), IfRefDouble=double, IfRefSingle=single, IsSigned=IsSigned1, NumBitsBase=NumBits1, NumBitsMult=1, NumBitsAdd=0, NumBitsAllowFinal=1:128, PropScalingMode=Inherit via propagation rule, PropScaling=2^-10, ValuesUsedBestPrec=[5 -7], SlopeBase=Slope1, SlopeMult=1, SlopeAdd=0, BiasBase=Bias1, BiasMult=1, BiasAdd=0}
      mask prompts: PropDataTypeMode "Simulink:masks:x1PropagatedDataType_MP"; PropDataType "Simulink:masks:x11PropagatedDataTypeegFixdt116Fixdtsingle_MP"; IfRefDouble "Simulink:masks:x11IfAnyReferenceInputIsDoubleOutputIs_MP"; IfRefSingle "Simulink:masks:x12IfAnyReferenceInputIsSingleOutputIs_MP"; IsSigned "Simulink:masks:x13IsSigned_MP"; NumBitsBase "Simulink:masks:x141NumberofBitsBase_MP"; NumBitsMult "Simulink:masks:x142NumberofBitsMultiplicativeAdjustment_MP"; NumBitsAdd "Simulink:masks:x143NumberofBitsAdditiveAdjustment_MP"; NumBitsAllowFinal "Simulink:masks:x144NumberofBitsAllowableFinalValues_MP"; PropScalingMode "Simulink:masks:x2PropagatedScaling_MP"; PropScaling "Simulink:masks:x21PropagatedScalingSlopeEg29OrSlopeBiasEg1253_MP"; ValuesUsedBestPrec "Simulink:masks:x21ValuesUsedToDetermineBestPrecisionScaling_MP"; SlopeBase "Simulink:masks:x211SlopeBase_MP"; SlopeMult "Simulink:masks:x212SlopeMultiplicativeAdjustment_MP"; SlopeAdd "Simulink:masks:x213SlopeAdditiveAdjustment_MP"; BiasBase "Simulink:masks:x221BiasBase_MP"; BiasMult "Simulink:masks:x222BiasMultiplicativeAdjustment_MP"; BiasAdd "Simulink:masks:x223BiasAdditiveAdjustment_MP"
      mask help: Simulink:masks:DataTypePropagation_MD
      mask init:
      | DblOver = 0;
      mask TypeOptions PropDataTypeMode: Simulink:masks:SpecifyViaDialog | Simulink:masks:InheritViaPropagationRule
      mask Callback PropDataTypeMode: fixptdialog(gcbh)
      mask Callback PropDataType: fixptdialog(gcbh)
      mask TypeOptions IfRefDouble: Simulink:masks:double | Simulink:masks:single
      mask TypeOptions IfRefSingle: Simulink:masks:double | Simulink:masks:single
      mask TypeOptions IsSigned: Simulink:masks:IsSigned1 | Simulink:masks:IsSigned2 | Simulink:masks:IsSigned1OrIsSigned2 | Simulink:masks:TRUE | Simulink:masks:FALSE
      mask TypeOptions NumBitsBase: NumBits1 | NumBits2 | max([NumBits1 NumBits2]) | min([NumBits1 NumBits2]) | NumBits1+NumBits2
      mask TypeOptions PropScalingMode: Simulink:masks:SpecifyViaDialog | Simulink:masks:InheritViaPropagationRule | Simulink:masks:ObtainViaBestPrecision
      mask Callback PropScalingMode: fixptdialog(gcbh)
      mask TypeOptions SlopeBase: Slope1 | Slope2 | max([Slope1 Slope2]) | min([Slope1 Slope2]) | Slope1*Slope2 | Slope1/Slope2 | PosRange1 | PosRange2 | max([PosRange1 PosRange2]) | min([PosRange1 PosRange2]) | PosRange1*PosRange2 | PosRange1/PosRange2
      mask TypeOptions BiasBase: Bias1 | Bias2 | max([Bias1 Bias2]) | min([Bias1 Bias2]) | Bias1*Bias2 | Bias1/Bias2 | Bias1+Bias2 | Bias1-Bias2
      mask Display:
      | port_label('Input',1,'Ref1');
      | port_label('Input',2,'Ref2');
      | port_label('Input',3,'Prop');
  LowerRelop1 : RelationalOperator  DisableCoverage=on  Operator=>  OutDataTypeStr=boolean  InputSameDT=off
  Switch : Switch  Criteria=u2 ~= 0  OutDataTypeStr=Inherit: Inherit via back propagation  ZeroCross=off  SaturateOnIntegerOverflow=off  InputSameDT=off
  Switch2 : Switch  Criteria=u2 ~= 0  OutMin=OutMin  OutMax=OutMax  OutDataTypeStr=Inherit: Inherit via back propagation  ZeroCross=off  SaturateOnIntegerOverflow=off  InputSameDT=off
  UpperRelop : RelationalOperator  DisableCoverage=on  Operator=<  OutDataTypeStr=boolean  InputSameDT=off
  y : Outport  OutMin=OutMin  OutMax=OutMax
  wires:
  up/1 -> Switch2/1, LowerRelop1/2
  u/1 -> Data Type Propagation/2, Data Type Propagation/1, LowerRelop1/1, Switch/3, UpperRelop/1
  lo/1 -> Switch/1, UpperRelop/2
  Switch/1 -> Data Type Duplicate/2, Switch2/3, Data Type Propagation/3
  Switch2/1 -> Data Type Duplicate/1, y/1
  LowerRelop1/1 -> Switch2/2
  UpperRelop/1 -> Switch/2

== system simModel2020/AutoPilot/InnerLoopAutopilot/Longitudinal Channel经度通道/AutoThrottle/AT Mode = 0,Recycle/Rate Limiter Dynamic with External IC and Autoreset for Change in IC/Subsystem ==
  WP Fly : Inport
  Compare To Constant : Subsystem  mask(Compare To Constant){relop=>=, const=0.5, OutDataTypeStr=boolean, ZeroCross=on}
      mask prompts: relop "Simulink:masks:Operator_MP"; const "Simulink:masks:ConstantValue_MP"; OutDataTypeStr "Simulink:masks:OutputDataType_MP"; ZeroCross "Simulink:masks:EnableZerocrossingDetection_MP"
      mask help: Simulink:masks:CompareToConstant_MD
      mask init:
      | blkName = gcb;
      | 
      | if strcmp(get_param(gcbh,'OutDataTypeStr'),'boolean')
      | 	setValue = 'boolean';
      | else
      | 	setValue = 'fixdt(0, 8)';
      | end
      | 
      | set_param([blkName,'/Compare'],'relop',relop, ...
      | 	'OutDataTypeStr', setValue, 'ZeroCross', ZeroCross);
      | 
      | str = [relop,' C']; %default
      | 
      | const_str = get_param(blkName, 'const');
      | const_val = str2num(const_str);
      | 
      | if isempty(const_val) %#ok<ST2NM>
      |     %Expression/Variable
      |     str = [relop, ' ', strtrim(const_str)];
      | else
      |     if length(const_val) == 1 
      |         if Simulink.data.isSupportedEnumClass(class(const_val))
      |             % Special Handling for Enumerations
      |             if Simulink.data.getEnumTypeInfo(class(const_val), 'AddClassNameToEnumNames')
      |                 str = [relop, ' ', strtrim(const_str)];
      |             else
      |                 str = [relop, ' ', char(const_val)];
      |             end
      |         elseif(isfloat(const_val) || isinteger(const_val) || islogical(const_val)) 
      |                 str = [relop, ' ', num2str(const_val)];
      |         end
      |     end
      | end
      mask TypeOptions relop: == | ~= | < | <= | >= | >
      mask TypeOptions OutDataTypeStr: Simulink:masks:uint8 | Simulink:masks:boolean
      mask Callback ZeroCross: sl('zeroCrossEnable', gcbh);
      mask Display: disp(str)
  Compare To Constant1 : Subsystem  mask(Compare To Constant){relop=<, const=0.5, OutDataTypeStr=boolean, ZeroCross=on}
      mask prompts: relop "Simulink:masks:Operator_MP"; const "Simulink:masks:ConstantValue_MP"; OutDataTypeStr "Simulink:masks:OutputDataType_MP"; ZeroCross "Simulink:masks:EnableZerocrossingDetection_MP"
      mask help: Simulink:masks:CompareToConstant_MD
      mask init: same as simModel2020/AutoPilot/InnerLoopAutopilot/Longitudinal Channel经度通道/AutoThrottle/AT Mode = 0,Recycle/Rate Limiter Dynamic with External IC and Autoreset for Change in IC/Subsystem/Compare To Constant
      mask TypeOptions relop: == | ~= | < | <= | >= | >
      mask TypeOptions OutDataTypeStr: Simulink:masks:uint8 | Simulink:masks:boolean
      mask Callback ZeroCross: sl('zeroCrossEnable', gcbh);
      mask Display: disp(str)
  Logical Operator : Logic  AllPortsSameDT=off  OutDataTypeStr=boolean
  Unit Delay : UnitDelay  SampleTime=-1  HasFrameUpgradeWarning=on
  Just Enab : Outport
  wires:
  WP Fly/1 -> Unit Delay/1, Compare To Constant/1(u)
  Compare To Constant/1(y) -> Logical Operator/1
  Compare To Constant1/1(y) -> Logical Operator/2
  Unit Delay/1 -> Compare To Constant1/1(u)
  Logical Operator/1 -> Just Enab/1

== system simModel2020/AutoPilot/InnerLoopAutopilot/Longitudinal Channel经度通道/AutoThrottle/AT Mode = 0,Recycle/Rate Limiter Dynamic with External IC and Autoreset for Change in IC/Unit Delay Resettable External IC ==
  note: Reset
  note: Initial Value
  u : Inport
  R : Inport  Port=2
  IC : Inport  Port=3
  FixPt Constant : Constant  DisableCoverage=on  Value=0  OutDataTypeStr=fixdt(0,8,0)
  FixPt Data Type Duplicate1 : DataTypeDuplicate  DisableCoverage=on  NumInputPorts=4
  FixPt Logical Operator : Logic  DisableCoverage=on  Operator=OR  AllPortsSameDT=off  OutDataTypeStr=fixdt(0, 8)
  FixPt Unit Delay1 : UnitDelay  DisableCoverage=on  InitialCondition=0.0  SampleTime=tsamp
  FixPt Unit Delay2 : UnitDelay  DisableCoverage=on  InitialCondition=1  SampleTime=tsamp  HasFrameUpgradeWarning=on
  Init : Switch  Criteria=u2 ~= 0  OutDataTypeStr=Inherit: Inherit via back propagation  ZeroCross=off  SaturateOnIntegerOverflow=off  InputSameDT=off
  Reset : Switch  Criteria=u2 ~= 0  OutDataTypeStr=Inherit: Inherit via back propagation  ZeroCross=off  SaturateOnIntegerOverflow=off  InputSameDT=off
  State Control : Subsystem  Description=Replaced Block  mask(Replaced Block){}
      mask help: This block has been replaced with an empty subsystem because it used functionality that is unavailable in Simulink R2014a.
      mask Display: fprintf('Replaced: %s\n','StateControl')
  y : Outport
  wires:
  FixPt Logical Operator/1 -> Init/2
  FixPt Unit Delay1/1 -> Init/3  "Xold"
  Init/1 -> y/1, FixPt Data Type Duplicate1/1
  FixPt Unit Delay2/1 -> FixPt Logical Operator/2
  FixPt Constant/1 -> FixPt Unit Delay2/1
  R/1 -> FixPt Logical Operator/1, Reset/2
  Reset/1 -> FixPt Unit Delay1/1, FixPt Data Type Duplicate1/2  "Xnew"
  u/1 -> Reset/3, FixPt Data Type Duplicate1/4
  IC/1 -> FixPt Data Type Duplicate1/3, Init/1, Reset/1

== system simModel2020/AutoPilot/InnerLoopAutopilot/Longitudinal Channel经度通道/AutoThrottle/AT Mode = 2,MCP Speed/Filter1/Subsystem ==
  In : Inport
  Enable : EnablePort  StatesWhenEnabling=reset
  " " : Outport  InitialOutput=0
  wires:
  In/1 -> " "/1

== system simModel2020/AutoPilot/InnerLoopAutopilot/Longitudinal Channel经度通道/AutoThrottle/AT Mode = 3,Throttle Control/Filter1/Subsystem ==
  In : Inport
  Enable : EnablePort  StatesWhenEnabling=reset
  " " : Outport  InitialOutput=0
  wires:
  In/1 -> " "/1

== system simModel2020/AutoPilot/InnerLoopAutopilot/Longitudinal Channel经度通道/AutoThrottle/AT Mode = 5,Idle/Filter1/Subsystem ==
  In : Inport
  Enable : EnablePort  StatesWhenEnabling=reset
  " " : Outport  InitialOutput=0
  wires:
  In/1 -> " "/1
